simulink model "Kajan_system_B_obtencion_datos"  (R2016a)
settings: Solver=VariableStepAuto  StartTime=0.0  StopTime=2500  RelTol=1e-3
values from neighbouring files (symbols this model uses):
  tm = 0.1    [ejemplodiscretro.m]
settings Model: Creator=Daniel  LastModifiedBy=Daniel

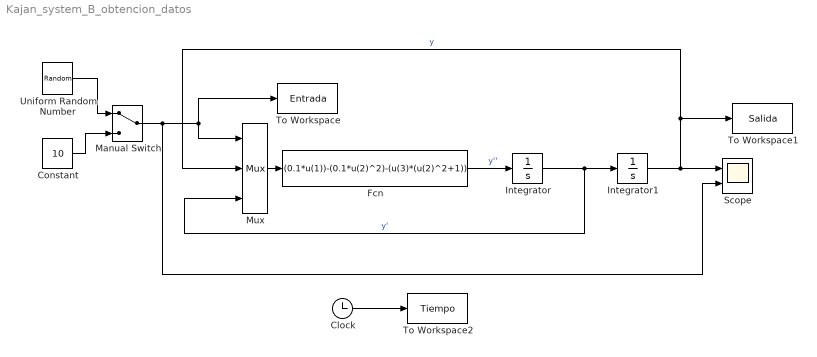
== system Kajan_system_B_obtencion_datos ==
  Clock : Clock
  Constant : Constant  Value=10
  "Fcn " : Fcn  Expr=(0.1*u(1))-(0.1*u(2)^2)-(u(3)*(u(2)^2+1))
  Integrator : Integrator
  Integrator1 : Integrator
  Manual Switch : ManualSwitch
  Mux : Mux  Inputs=3
  Scope : Scope  NumInputPorts=2
  To Workspace : ToWorkspace  VariableName=Entrada  SampleTime=tm
  To Workspace1 : ToWorkspace  VariableName=Salida  SampleTime=tm
  To Workspace2 : ToWorkspace  VariableName=Tiempo  SampleTime=tm
  Uniform Random Number : UniformRandomNumber  Minimum=0  Maximum=10  SampleTime=100
  wires:
  "Fcn "/1 -> Integrator/1  "y''"
  Integrator/1 -> Integrator1/1, Mux/3  "y'"
  Mux/1 -> "Fcn "/1
  Integrator1/1 -> Mux/2, To Workspace1/1, Scope/1  "y"
  Uniform Random Number/1 -> Manual Switch/1
  Manual Switch/1 -> To Workspace/1, Mux/1, Scope/2
  Constant/1 -> Manual Switch/2
  Clock/1 -> To Workspace2/1
